simulink model "simulation_ex6_2"  (R2023a)
settings: Solver=VariableStepAuto  StartTime=0.0  StopTime=10  RelTol=1e-3
settings Model: Creator=vigro  LastModifiedBy=vigro
settings DataIOCC: ReturnWorkspaceOutputs=off

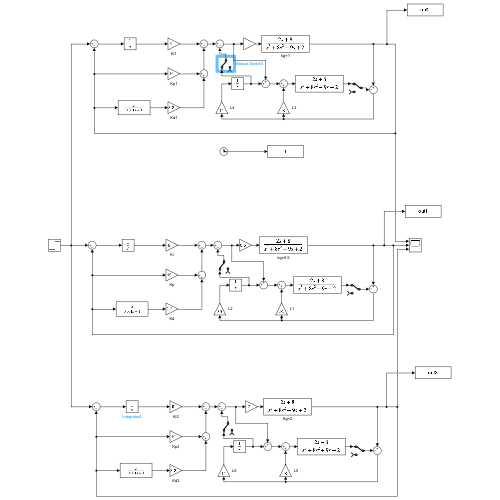
[thumbnail: Simulink's stored preview of the top-level diagram]
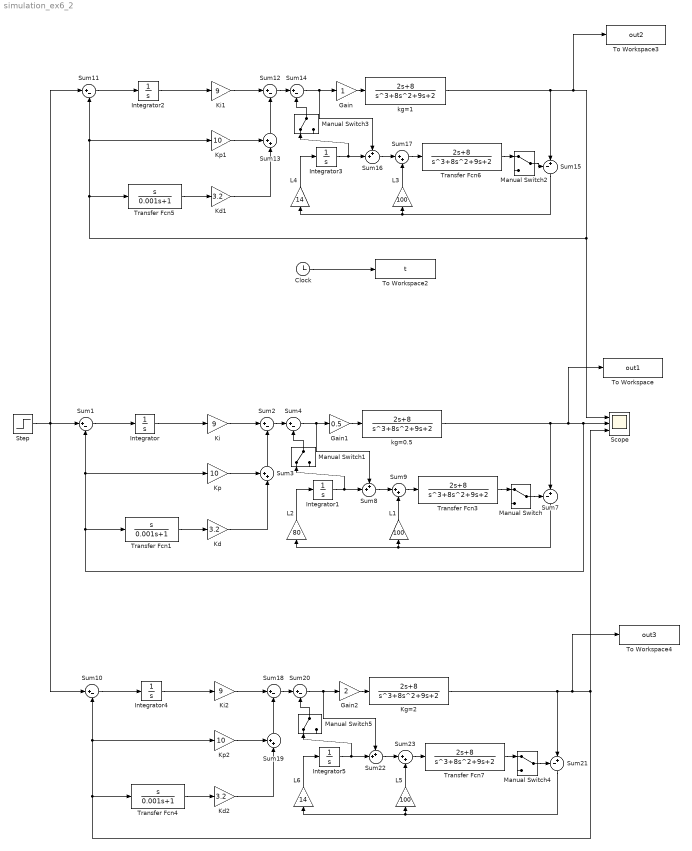
== system simulation_ex6_2 ==
  Clock : Clock
  Gain : Gain
  Gain1 : Gain  Gain=0.5
  Gain2 : Gain  Gain=2
  Integrator{,1..5} (6 alike) : Integrator
  Kd : Gain  Gain=3.2
  Kd1 : Gain  Gain=3.2
  Kd2 : Gain  Gain=3.2
  Kg=2 : TransferFcn  Numerator=[2 8]  Denominator=[1 8 9 2]
  Ki : Gain  Gain=9
  Ki1 : Gain  Gain=9
  Ki2 : Gain  Gain=9
  Kp : Gain  Gain=10
  Kp1 : Gain  Gain=10
  Kp2 : Gain  Gain=10
  L1 : Gain  Gain=100
  L2 : Gain  Gain=80
  L3 : Gain  Gain=100
  L4 : Gain  Gain=14
  L5 : Gain  Gain=100
  L6 : Gain  Gain=14
  Manual Switch{,1..5} (6 alike) : ManualSwitch
  Scope : Scope  NumInputPorts=3
  Step : Step  Time=2  SampleTime=0
  Sum{1..2,4,10..12,14,18,20} (9 alike) : Sum  Inputs=|+-
  Sum{3,8,13,16,19,22} (6 alike) : Sum  Inputs=++|
  Sum15 : Sum  Inputs=-+|
  Sum17 : Sum  Inputs=|++
  Sum21 : Sum  Inputs=-+|
  Sum23 : Sum  Inputs=|++
  Sum7 : Sum  Inputs=-+|
  Sum9 : Sum  Inputs=|++
  To Workspace : ToWorkspace  VariableName=out1  SaveFormat=Timeseries  SampleTime=-1
  To Workspace2 : ToWorkspace  VariableName=t  SaveFormat=Timeseries  SampleTime=-1
  To Workspace3 : ToWorkspace  VariableName=out2  SaveFormat=Timeseries  SampleTime=-1
  To Workspace4 : ToWorkspace  VariableName=out3  SaveFormat=Timeseries  SampleTime=-1
  Transfer Fcn1 : TransferFcn  Numerator=[1 0]  Denominator=[0.001 1]
  Transfer Fcn3 : TransferFcn  Numerator=[2 8]  Denominator=[1 8 9 2]
  Transfer Fcn4 : TransferFcn  Numerator=[1 0]  Denominator=[0.001 1]
  Transfer Fcn5 : TransferFcn  Numerator=[1 0]  Denominator=[0.001 1]
  Transfer Fcn6 : TransferFcn  Numerator=[2 8]  Denominator=[1 8 9 2]
  Transfer Fcn7 : TransferFcn  Numerator=[2 8]  Denominator=[1 8 9 2]
  kg=0.5 : TransferFcn  Numerator=[2 8]  Denominator=[1 8 9 2]
  kg=1 : TransferFcn  Numerator=[2 8]  Denominator=[1 8 9 2]
  wires:
  Step/1 -> Sum10/1, Sum11/1, Sum1/1
  Sum1/1 -> Integrator/1
  Integrator/1 -> Ki/1
  Ki/1 -> Sum2/1
  Gain1/1 -> kg=0.5/1
  Kp/1 -> Sum3/1
  Sum3/1 -> Sum2/2
  Kd/1 -> Sum3/2
  Transfer Fcn1/1 -> Kd/1
  kg=0.5/1 -> Transfer Fcn1/1, Kp/1, Sum1/2, Scope/2, To Workspace/1, Sum7/2
  Sum2/1 -> Sum4/1
  Sum4/1 -> Sum8/1, Gain1/1
  Clock/1 -> To Workspace2/1
  Transfer Fcn3/1 -> Manual Switch/1
  Manual Switch/1 -> Sum7/1
  Integrator1/1 -> Manual Switch1/1, Sum8/2
  L2/1 -> Integrator1/1
  Sum7/1 -> L2/1, L1/1
  Manual Switch1/1 -> Sum4/2
  Sum9/1 -> Transfer Fcn3/1
  Sum8/1 -> Sum9/1
  L1/1 -> Sum9/2
  Sum16/1 -> Sum17/1
  L3/1 -> Sum17/2
  Sum15/1 -> L4/1, L3/1
  Manual Switch3/1 -> Sum14/2
  Manual Switch2/1 -> Sum15/1
  Transfer Fcn6/1 -> Manual Switch2/1
  L4/1 -> Integrator3/1
  Sum12/1 -> Sum14/1
  kg=1/1 -> Scope/1, Transfer Fcn5/1, Kp1/1, Sum11/2, To Workspace3/1, Sum15/2
  Gain/1 -> kg=1/1
  Sum17/1 -> Transfer Fcn6/1
  Sum13/1 -> Sum12/2
  Integrator2/1 -> Ki1/1
  Kp1/1 -> Sum13/1
  Sum11/1 -> Integrator2/1
  Integrator3/1 -> Manual Switch3/1, Sum16/2
  Transfer Fcn5/1 -> Kd1/1
  Kd1/1 -> Sum13/2
  Sum14/1 -> Gain/1, Sum16/1
  Ki1/1 -> Sum12/1
  Sum22/1 -> Sum23/1
  Sum21/1 -> L6/1, L5/1
  Sum20/1 -> Gain2/1, Sum22/1
  Ki2/1 -> Sum18/1
  Integrator5/1 -> Manual Switch5/1, Sum22/2
  Sum19/1 -> Sum18/2
  Sum23/1 -> Transfer Fcn7/1
  Manual Switch5/1 -> Sum20/2
  Sum10/1 -> Integrator4/1
  Integrator4/1 -> Ki2/1
  Gain2/1 -> Kg=2/1
  Manual Switch4/1 -> Sum21/1
  Transfer Fcn4/1 -> Kd2/1
  Sum18/1 -> Sum20/1
  Kg=2/1 -> Scope/3, Transfer Fcn4/1, Kp2/1, Sum10/2, To Workspace4/1, Sum21/2
  Kp2/1 -> Sum19/1
  L5/1 -> Sum23/2
  L6/1 -> Integrator5/1
  Kd2/1 -> Sum19/2
  Transfer Fcn7/1 -> Manual Switch4/1
